simulink model "lab_1"  (R2021b)
settings: Solver=VariableStepAuto  StartTime=0.0  StopTime=15  MaxStep=1e-2  RelTol=1e-3
values from neighbouring files (symbols this model uses):
  a = 0.5    [env_lab_1.m]
  am = -5    [env_lab_1.m]
  b = 1    [env_lab_1.m]
  bm = 5    [env_lab_1.m]
  ga = 100    [env_lab_1.m]
  gb = ga    (= 100)    [env_lab_1.m]
  P = 2    [env_lab_1.m]
undefined symbols (not defined in the file or in its folder): as, au, bs, bu
settings Model: Creator=79159  LastModifiedBy=79159

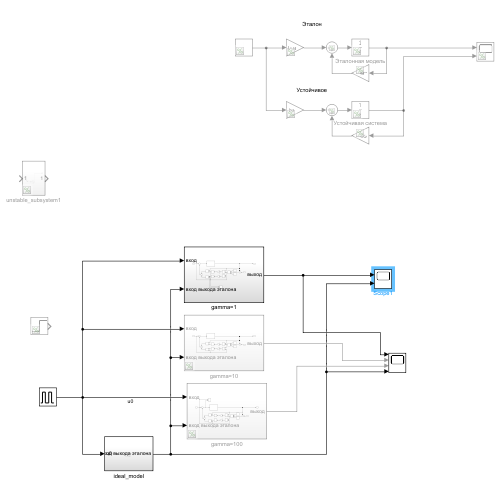
[thumbnail: Simulink's stored preview of the top-level diagram]
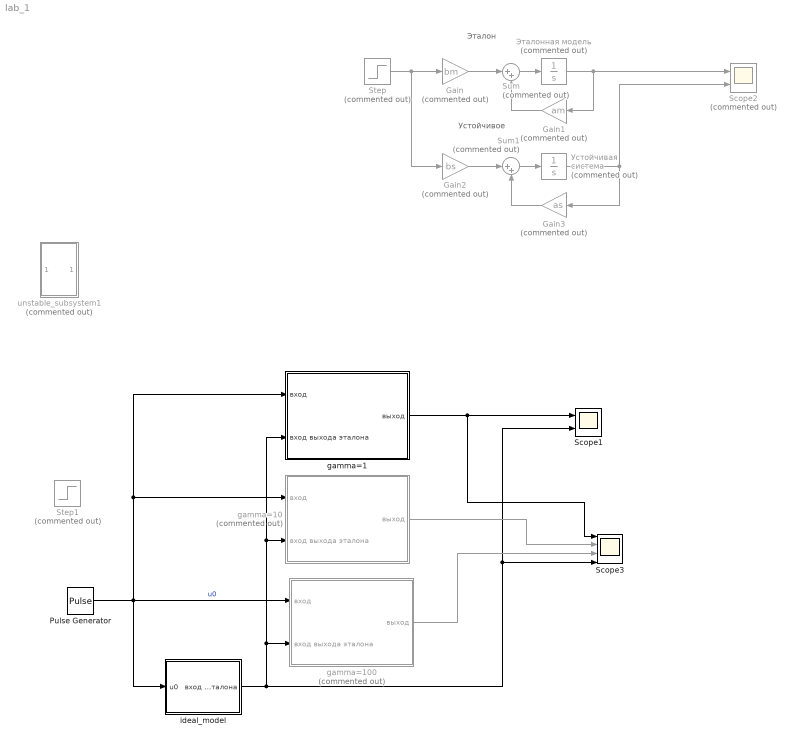
== system lab_1 ==
  note: Устойчивое
  note: Эталон
  Gain : Gain  Commented=on  Gain=bm
  Gain1 : Gain  Commented=on  Gain=am
  Gain2 : Gain  Commented=on  Gain=bs
  Gain3 : Gain  Commented=on  Gain=as
  Pulse Generator : DiscretePulseGenerator  PulseType=Time based  Period=5  PulseWidth=50
  Scope1 : Scope  NumInputPorts=2
  Scope2 : Scope  Commented=on  NumInputPorts=2
  Scope3 : Scope  NumInputPorts=4
  Step : Step  Commented=on  Time=0  SampleTime=0
  Step1 : Step  Commented=on  Time=0  SampleTime=0
  Sum : Sum  Commented=on  Inputs=|++
  Sum1 : Sum  Commented=on  Inputs=|++
  gamma=1 : Subsystem
  gamma=10 : Subsystem  Commented=on
  gamma=100 : Subsystem  Commented=on
  ideal_model : Subsystem
  unstable_subsystem1 : Subsystem  Commented=on
  Устойчивая система : Integrator  Commented=on
  Эталонная модель : Integrator  Commented=on
  wires:
  Gain/1 -> Sum/1
  Sum/1 -> Эталонная модель/1
  Step/1 -> Gain2/1, Gain/1
  Gain1/1 -> Sum/2
  Эталонная модель/1 -> Scope2/1, Gain1/1
  Gain3/1 -> Sum1/2
  Sum1/1 -> Устойчивая система/1
  Gain2/1 -> Sum1/1
  Устойчивая система/1 -> Scope2/2, Gain3/1
  Pulse Generator/1 -> gamma=1/1(вход), gamma=10/1(вход), gamma=100/1(вход), ideal_model/1(u0)  "u0"
  ideal_model/1(вход выхода эталона) -> Scope1/2, Scope3/4, gamma=1/2(вход выхода эталона), gamma=10/2(вход выхода эталона), gamma=100/2(вход выхода эталона)
  gamma=100/1(выход) -> Scope3/3
  gamma=10/1(выход) -> Scope3/2
  gamma=1/1(выход) -> Scope1/1, Scope3/1

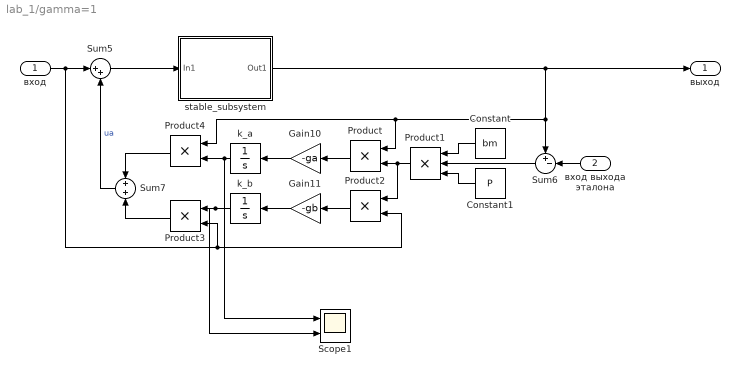
== system lab_1/gamma=1 ==
  вход : Inport
  вход выхода эталона : Inport  Port=2
  Constant : Constant  Value=bm
  Constant1 : Constant  Value=P
  Gain10 : Gain  Gain=-ga
  Gain11 : Gain  Gain=-gb
  Product{,2..4} (4 alike) : Product
  Product1 : Product  Inputs=3
  Scope1 : Scope  NumInputPorts=2
  Sum5 : Sum  Inputs=|++
  Sum6 : Sum  Inputs=+-|
  Sum7 : Sum
  k_a : Integrator
  k_b : Integrator
  stable_subsystem : Subsystem
  выход : Outport
  wires:
  Product3/1 -> Sum7/2
  Sum6/1 -> Product1/2
  Gain10/1 -> k_a/1
  k_b/1 -> Scope1/2, Product3/1
  Sum7/1 -> Sum5/2  "ua"
  k_a/1 -> Product4/2, Scope1/1
  вход/1 -> Product2/2, Product3/2, Sum5/1
  stable_subsystem/1(Out1) -> выход/1, Sum6/1, Product/1, Product4/1
  Constant/1 -> Product1/1
  Product2/1 -> Gain11/1
  Product4/1 -> Sum7/1
  Product/1 -> Gain10/1
  Gain11/1 -> k_b/1
  Sum5/1 -> stable_subsystem/1(In1)
  Product1/1 -> Product2/1, Product/2
  Constant1/1 -> Product1/3
  вход выхода эталона/1 -> Sum6/2

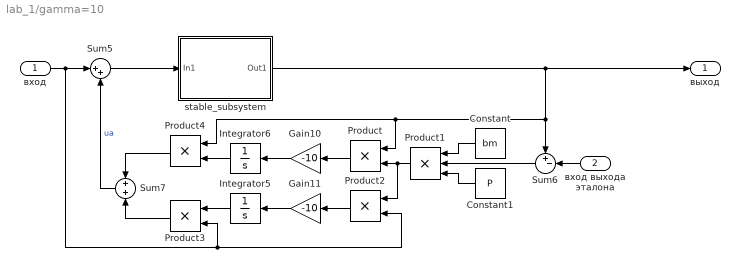
== system lab_1/gamma=10 ==
  вход : Inport
  вход выхода эталона : Inport  Port=2
  Constant : Constant  Value=bm
  Constant1 : Constant  Value=P
  Gain10 : Gain  Gain=-10
  Gain11 : Gain  Gain=-10
  Integrator5 : Integrator
  Integrator6 : Integrator
  Product{,2..4} (4 alike) : Product
  Product1 : Product  Inputs=3
  Sum5 : Sum  Inputs=|++
  Sum6 : Sum  Inputs=+-|
  Sum7 : Sum
  stable_subsystem : Subsystem
  выход : Outport
  wires:
  вход выхода эталона/1 -> Sum6/2
  Constant1/1 -> Product1/3
  Product1/1 -> Product/2, Product2/1
  Sum5/1 -> stable_subsystem/1(In1)
  Gain11/1 -> Integrator5/1
  Product/1 -> Gain10/1
  Product4/1 -> Sum7/1
  Product2/1 -> Gain11/1
  Constant/1 -> Product1/1
  stable_subsystem/1(Out1) -> Product4/1, Product/1, Sum6/1, выход/1
  вход/1 -> Sum5/1, Product3/2, Product2/2
  Integrator6/1 -> Product4/2
  Sum7/1 -> Sum5/2  "ua"
  Integrator5/1 -> Product3/1
  Gain10/1 -> Integrator6/1
  Sum6/1 -> Product1/2
  Product3/1 -> Sum7/2

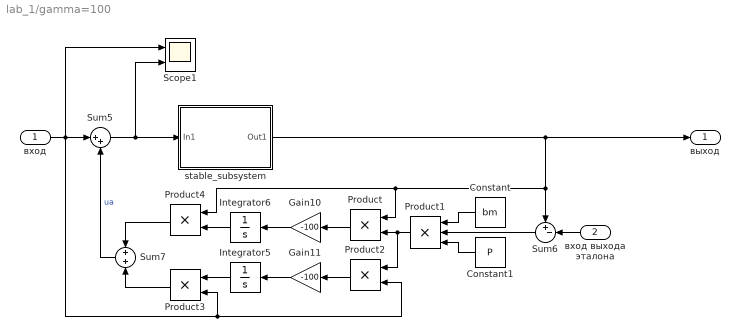
== system lab_1/gamma=100 ==
  вход : Inport
  вход выхода эталона : Inport  Port=2
  Constant : Constant  Value=bm
  Constant1 : Constant  Value=P
  Gain10 : Gain  Gain=-100
  Gain11 : Gain  Gain=-100
  Integrator5 : Integrator
  Integrator6 : Integrator
  Product{,2..4} (4 alike) : Product
  Product1 : Product  Inputs=3
  Scope1 : Scope  NumInputPorts=2
  Sum5 : Sum  Inputs=|++
  Sum6 : Sum  Inputs=+-|
  Sum7 : Sum
  stable_subsystem : Subsystem
  выход : Outport
  wires:
  Product3/1 -> Sum7/2
  Sum6/1 -> Product1/2
  Gain10/1 -> Integrator6/1
  Integrator5/1 -> Product3/1
  Sum7/1 -> Sum5/2  "ua"
  Integrator6/1 -> Product4/2
  вход/1 -> Scope1/1, Product2/2, Product3/2, Sum5/1
  stable_subsystem/1(Out1) -> выход/1, Sum6/1, Product/1, Product4/1
  Constant/1 -> Product1/1
  Product2/1 -> Gain11/1
  Product4/1 -> Sum7/1
  Product/1 -> Gain10/1
  Gain11/1 -> Integrator5/1
  Sum5/1 -> Scope1/2, stable_subsystem/1(In1)
  Product1/1 -> Product2/1, Product/2
  Constant1/1 -> Product1/3
  вход выхода эталона/1 -> Sum6/2

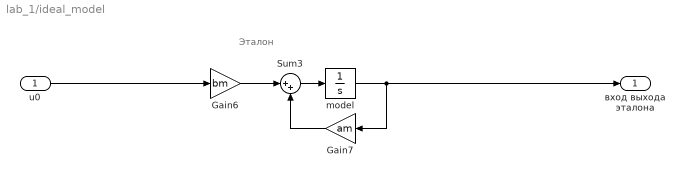
== system lab_1/ideal_model ==
  note: Эталон
  u0 : Inport
  Gain6 : Gain  Gain=bm
  Gain7 : Gain  Gain=am
  Sum3 : Sum  Inputs=|++
  model : Integrator
  вход выхода эталона : Outport
  wires:
  model/1 -> вход выхода эталона/1, Gain7/1
  Sum3/1 -> model/1
  Gain6/1 -> Sum3/1
  Gain7/1 -> Sum3/2
  u0/1 -> Gain6/1

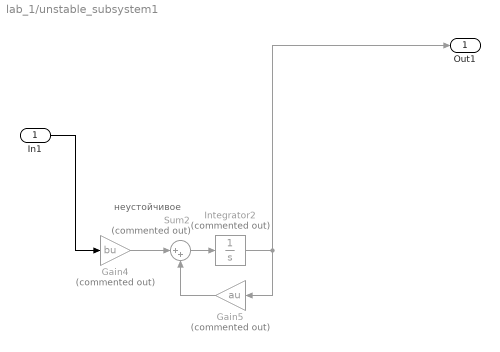
== system lab_1/unstable_subsystem1 ==
  note: неустойчивое
  In1 : Inport
  Gain4 : Gain  Commented=on  Gain=bu
  Gain5 : Gain  Commented=on  Gain=au
  Integrator2 : Integrator  Commented=on
  Sum2 : Sum  Commented=on  Inputs=|++
  Out1 : Outport
  wires:
  Gain4/1 -> Sum2/1
  Sum2/1 -> Integrator2/1
  In1/1 -> Gain4/1
  Gain5/1 -> Sum2/2
  Integrator2/1 -> Gain5/1, Out1/1

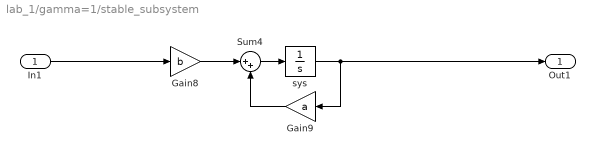
== system lab_1/gamma=1/stable_subsystem ==
  In1 : Inport
  Gain8 : Gain  Gain=b
  Gain9 : Gain  Gain=a
  Sum4 : Sum  Inputs=|++
  sys : Integrator
  Out1 : Outport
  wires:
  In1/1 -> Gain8/1
  sys/1 -> Out1/1, Gain9/1
  Gain8/1 -> Sum4/1
  Sum4/1 -> sys/1
  Gain9/1 -> Sum4/2

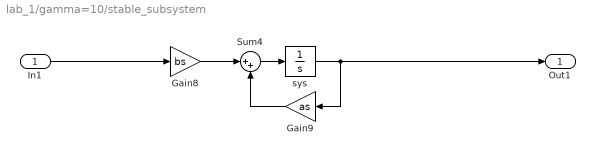
== system lab_1/gamma=10/stable_subsystem ==
  In1 : Inport
  Gain8 : Gain  Gain=bs
  Gain9 : Gain  Gain=as
  Sum4 : Sum  Inputs=|++
  sys : Integrator
  Out1 : Outport
  wires:
  Gain9/1 -> Sum4/2
  Sum4/1 -> sys/1
  Gain8/1 -> Sum4/1
  sys/1 -> Gain9/1, Out1/1
  In1/1 -> Gain8/1

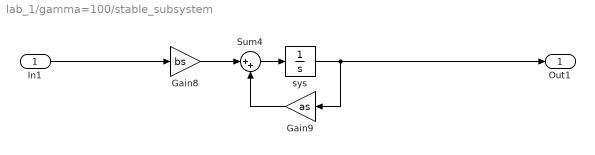
== system lab_1/gamma=100/stable_subsystem ==
  In1 : Inport
  Gain8 : Gain  Gain=bs
  Gain9 : Gain  Gain=as
  Sum4 : Sum  Inputs=|++
  sys : Integrator
  Out1 : Outport
  wires:
  In1/1 -> Gain8/1
  sys/1 -> Out1/1, Gain9/1
  Gain8/1 -> Sum4/1
  Sum4/1 -> sys/1
  Gain9/1 -> Sum4/2
